simulink model "controller"  (R2020a)
settings: Solver=VariableStepAuto  StartTime=0.0  StopTime=10  RelTol=1e-3
undefined symbols (not defined in the file or in its folder): Angular, Linear
libraries: robotlib x3
settings Model: Creator=javier  LastModifiedBy=javier

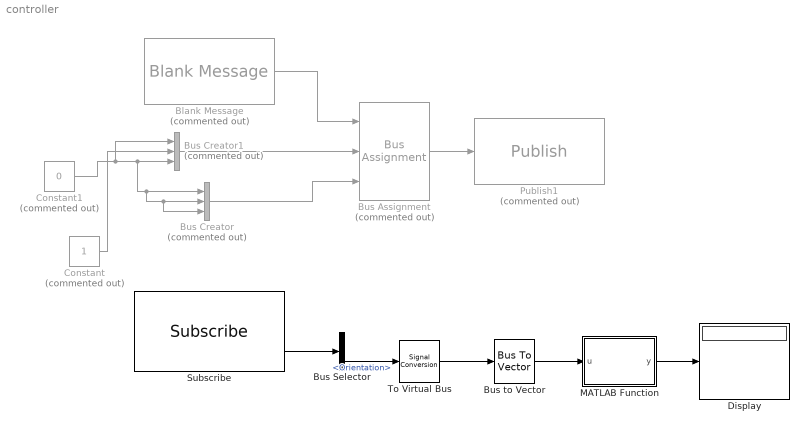
== system controller ==
  Blank Message : robotlib/Blank Message  Commented=on  messageClass=Message  entityType=geometry_msgs/Twist  messageType=geometry_msgs/Twist  SampleTime=inf
  Bus Assignment : BusAssignment  Commented=on  AssignedSignals=Linear,Angular
  Bus Creator : BusCreator  Commented=on  Inputs=3
  Bus Creator1 : BusCreator  Commented=on  Inputs=3
  Bus Selector : BusSelector  OutputSignals=Pose.Pose.Position,Pose.Pose.Orientation
  Bus to Vector : BusToVector
  Constant : Constant  Commented=on
  Constant1 : Constant  Commented=on  Value=0
  Display : Display
  MATLAB Function : MATLAB Function  TreatAsAtomicUnit=on
  Publish1 : robotlib/Publish  Commented=on  topicSource=Select from ROS network  topic=/kh4_diff_drive_controller/cmd_vel  messageType=geometry_msgs/Twist  messageQueueLength=105
  Subscribe : robotlib/Subscribe  topicSource=Select from ROS network  topic=/kh4_diff_drive_controller/odom  messageType=nav_msgs/Odometry  sampleTime=-1  messageQueueLength=1
  To Virtual Bus : SignalConversion  ConversionOutput=Virtual bus  OverrideOpt=off
  wires:
  Bus Creator/1 -> Bus Assignment/3
  Bus Creator1/1 -> Bus Assignment/2
  Blank Message/1 -> Bus Assignment/1
  Constant1/1 -> Bus Creator1/1, Bus Creator/3, Bus Creator/2, Bus Creator/1, Bus Creator1/3
  Subscribe/2 -> Bus Selector/1
  Constant/1 -> Bus Creator1/2
  MATLAB Function/1(y) -> Display/1
  Bus Assignment/1 -> Publish1/1
  Bus to Vector/1 -> MATLAB Function/1(u)
  To Virtual Bus/1 -> Bus to Vector/1
  Bus Selector/2 -> To Virtual Bus/1  "<Orientation>"

== matlab function controller/MATLAB Function ==
  data: u input; y output
function y = fcn(u)

y = quat2eul(u');
